simulink model "Balance_DualGyro_150302"  (R2014a)
settings: Solver=FixedStepDiscrete  SolverMode=SingleTasking  StartTime=0.0  StopTime=inf  FixedStep=TS  RelTol=1e-3
undefined symbols (not defined in the file or in its folder): DiscIntNeverNeededParam, ES, GS, KLQR, Rw, TS
libraries: arduinolib x7, simulink x4
settings Model: FPTRunName=FPA_Reference  SimulationMode=external  ExtModeTrigDuration=2  Creator=Alec  LastModifiedBy=Brian
settings OptimizationCC: ExpressionDepthLimit=2147483647  OptimizeModelRefInitCode=on  LifeSpan=1
settings DebuggingCC: UnderspecifiedInitializationDetection=Classic  SolverPrmCheckMsg=none  StateNameClashWarn=warning
settings HardwareCC: ProdBitPerInt=16  ProdBitPerPointer=8  ProdIntDivRoundTo=Zero  ProdEndianess=LittleEndian  ProdWordSize=8  ProdHWDeviceType=Atmel->AVR
settings RTWCC: SystemTargetFile=realtime.tlc  GenerateMakefile=off  TemplateMakefile=realtime.tmf  Description=Real-Time Toolbox  RTWVerbose=off  ProcessScript=realtime_make_rtw_hook
settings CodeAppCC: CustomSymbolStrType=$N$R$M  InternalIdentifier=Classic
settings STFCustomTargetCC: TargetLibSuffix=.a  GenerateSampleERTMain=on  ConcurrentExecutionCompliant=off  GeneratePreprocessorConditionals=Use local settings  ERTCustomFileBanners=on  SupportNonInlinedSFcns=off  SupportVariableSizeSignals=on  MATLABClassNameForMDSCustomization=Simulink.SoftwareTarget.ERTCustomization  GRTInterface=off  SystemTargetFile=realtime.tlc
settings ERTTargetCC: CombineOutputUpdateFcns=off  SupportContinuousTime=on  SupportVariableSizeSignals=on  ExtModeTransport=3  ExtModeMexFile=ext_serial_win32_comm  ExtModeMexArgs=0 6 115200  ERTSrcFileBannerTemplate=realtime_code_template.cgt  ERTHdrFileBannerTemplate=realtime_code_template.cgt  ERTDataSrcFileTemplate=realtime_code_template.cgt  ERTDataHdrFileTemplate=realtime_code_template.cgt  ERTCustomFileTemplate=realtime_file_process.tlc

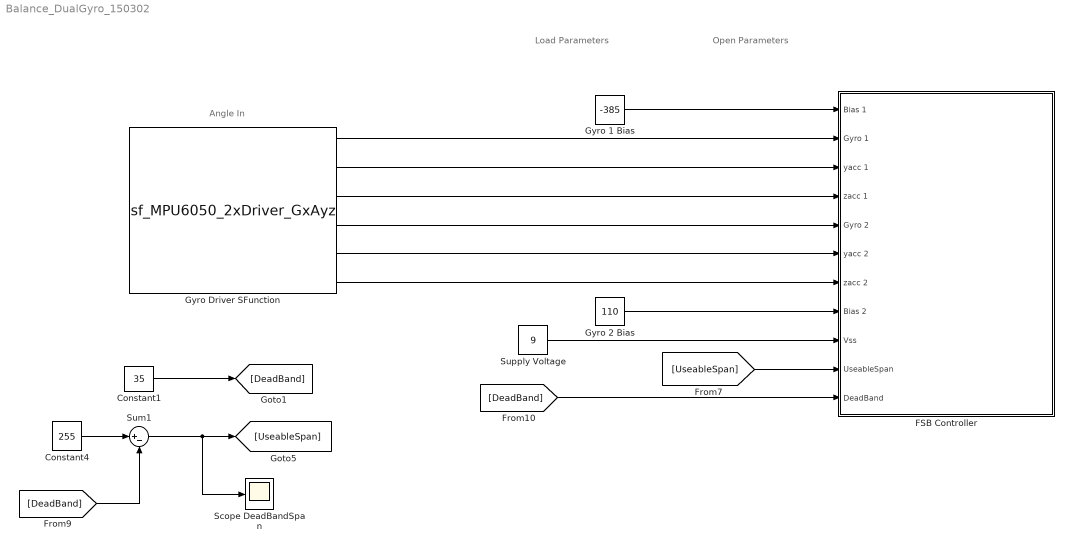
== system Balance_DualGyro_150302 ==
  note: Load Parameters
  note: Open Parameters
  note: Angle In
  Constant1 : Constant  Value=35
  Constant4 : Constant  Value=255
  FSB Controller : Subsystem
  Gyro 1 Bias : Constant  Value=-385
  Gyro 2 Bias : Constant  Value=110
  Gyro Driver SFunction : S-Function  InitFcn=try, set_param(gcb,'FunctionName','sf_MPU6050_2xDriver_GxAyz'), end  FunctionName=sf_MPU6050_2xDriver_GxAyz  SFunctionModules=sf_MPU6050_2xDriver_GxAyz_wrapper  EnableBusSupport=off  mask(S-Function Builder){}
      mask help: Simulink:masks:SFunctionBuilder_MD
      mask init:
      | val = [[.9  0.75 0.75 1 1 .9 .9 1]',[1 1 0.75 0.75 .9 .9 1 .9]'];try , sys = get_param(gcb,'SfunBuilderFcnName');if isempty(sys), sys = get_param(gcb,'FunctionName'); end,catch, sys = get_param(gcb,'FunctionName'); end
      settings: CopyFcn=set_param(gcbh,'LinkStatus','none')  PreSaveFcn=try, set_param(gcb,'FunctionName','sf_MPU6050_2xDriver_GxAyz'), end  OpenFcn=sfunctionwizard(gcbh)
      mask Display: plot(val(:,1),val(:,2)),disp(sys), port_label('output',1,'x_vel'), port_label('output',2,'y_acc'), port_label('output',3,'z_acc'), port_label('output',4,'x_vel_2'), port_label('output',5,'y_acc_2'), port_label('output',6,'z_acc_2')
  Scope DeadBandSpan : Scope
      settings: YMin=205  YMax=205  SaveName=ScopeData5
  Sum1 : Sum  Inputs=|+-
  Supply Voltage : Constant  Value=9
  wires:
  Gyro Driver SFunction/3 -> FSB Controller/4("zacc 1 ")
  Gyro 1 Bias/1 -> FSB Controller/1(Bias 1)
  Constant1/1 -> [DeadBand]
  Constant4/1 -> Sum1/1
  [DeadBand] -> Sum1/2
  Sum1/1 -> Scope DeadBandSpan/1, [UseableSpan]
  [DeadBand] -> FSB Controller/11(DeadBand)
  Supply Voltage/1 -> FSB Controller/9(Vss)
  Gyro Driver SFunction/2 -> FSB Controller/3("yacc 1 ")
  [UseableSpan] -> FSB Controller/10(UseableSpan)
  Gyro 2 Bias/1 -> FSB Controller/8(Bias 2)
  Gyro Driver SFunction/4 -> FSB Controller/5(Gyro 2)
  Gyro Driver SFunction/5 -> FSB Controller/6(yacc 2)
  Gyro Driver SFunction/6 -> FSB Controller/7(zacc 2)
  Gyro Driver SFunction/1 -> FSB Controller/2(Gyro 1)

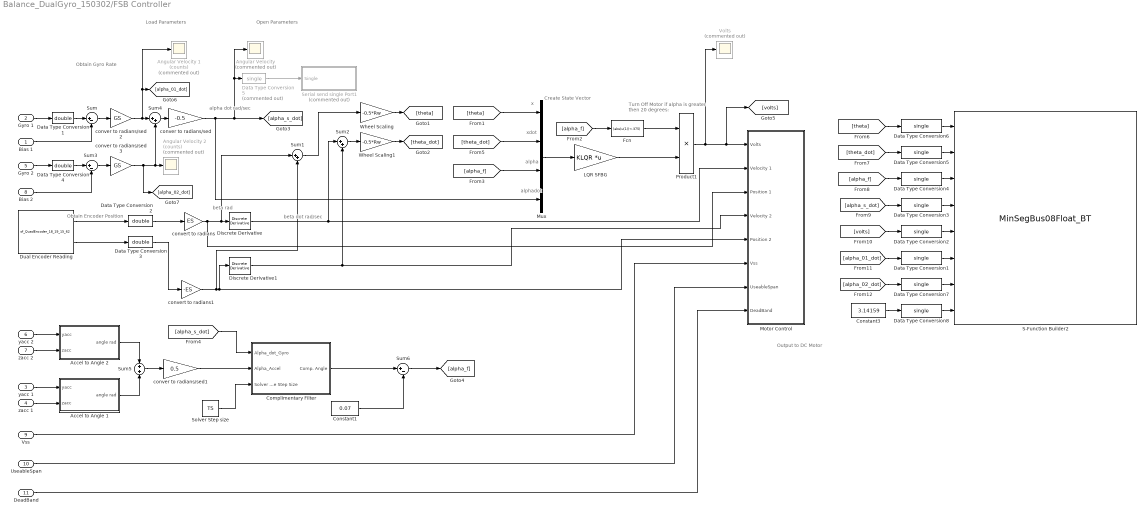
== system Balance_DualGyro_150302/FSB Controller ==
  note: Turn Off Motor if alpha is
      | greater then 20 degrees:
  note: Output to DC Motor
  note: Create State Vector
  note: Obtain Encoder Position
  note: Obtain Gyro Rate
  note: xdot
  note: x
  note: beta
      | rad
  note: alpha dot
      | rad/sec
  note: beta dot
      | rad/sec
  note: alpha
  note: alphadot
  note: Load Parameters
  note: Open Parameters
  Bias 1 : Inport
  Gyro 1 : Inport  Port=2
  "yacc 1 " : Inport  Port=3
  "zacc 1 " : Inport  Port=4
  Gyro 2 : Inport  Port=5
  yacc 2 : Inport  Port=6
  zacc 2 : Inport  Port=7
  Bias 2 : Inport  Port=8
  Vss : Inport  Port=9
  UseableSpan : Inport  Port=10
  DeadBand : Inport  Port=11
  Accel to Angle 1 : Subsystem
  Accel to Angle 2 : Subsystem
  Angular Velocity : Scope  Commented=on
      settings: YMin=-0.25  YMax=0.175
  Angular Velocity 1 (counts) : Scope  Commented=on
      settings: YMin=100  YMax=500  SaveName=ScopeData13
  Angular Velocity 2 (counts) : Scope  Commented=on
      settings: YMin=100  YMax=500  SaveName=ScopeData14
  Complimentary Filter : Subsystem
  Constant1 : Constant  Value=0.07
  Constant3 : Constant  Value=3.14159
  Data Type Conversion{1..4} (4 alike) : DataTypeConversion  OutDataTypeStr=double
  Data Type Conversion5 : DataTypeConversion  Commented=on  OutDataTypeStr=single
  Data Type Conversion{1..8} (8 alike) : DataTypeConversion  OutDataTypeStr=single
  Discrete Derivative : simulink/Discrete/Discrete Derivative  gainval=1.0  ICPrevScaledInput=0.0  InputProcessing=Inherited  OutMin=[]  OutMax=[]  OutDataType=fixdt(1, 16)  OutScaling=2^-10  DoSatur=off
  Discrete Derivative1 : simulink/Discrete/Discrete Derivative  gainval=1.0  ICPrevScaledInput=0.0  InputProcessing=Inherited  OutMin=[]  OutMax=[]  OutDataType=fixdt(1, 16)  OutScaling=2^-10  DoSatur=off
  Dual Encoder Reading : S-Function  InitFcn=try, set_param(gcb,'FunctionName','sf_QuadEncoder_18_19_15_62'), end  FunctionName=sf_QuadEncoder_18_19_15_62  Parameters=uint8([0 1]),uint8([18 62]),uint8([19 15])  SFunctionModules=sf_QuadEncoder_18_19_15_62_wrapper  EnableBusSupport=off  mask(S-Function Builder){}
      mask init: same as Balance_DualGyro_150302/Gyro Driver SFunction
      settings: CopyFcn=set_param(gcbh,'LinkStatus','none')  PreSaveFcn=try, set_param(gcb,'FunctionName','sf_QuadEncoder_18_19_15_62'), end  OpenFcn=sfunctionwizard(gcbh)
      mask Display: plot(val(:,1),val(:,2)),disp(sys), port_label('output',1,'pos1'), port_label('output',2,'pos2')
  Fcn : Fcn  Expr=(abs(u(1))<.375)
  LQR SFBG : Gain  Gain=KLQR  Multiplication=Matrix(K*u)
  Motor Control : Subsystem
  Mux : Mux
  Product1 : Product  RndMeth=Zero
  S-Function Builder2 : S-Function  InitFcn=try, set_param(gcb,'FunctionName','MinSegBus08Float_BT'), end  FunctionName=MinSegBus08Float_BT  Parameters=int8(4)  SFunctionModules=MinSegBus08Float_BT_wrapper  EnableBusSupport=off  mask(S-Function Builder){}
      mask help: Simulink:masks:SFunctionBuilder_MD
      mask init: same as Balance_DualGyro_150302/Gyro Driver SFunction
      settings: CopyFcn=set_param(gcbh,'LinkStatus','none')  PreSaveFcn=try, set_param(gcb,'FunctionName','MinSegBus08Float_BT'), end  OpenFcn=sfunctionwizard(gcbh)
      mask Display: plot(val(:,1),val(:,2)),disp(sys), port_label('input',1,'float_01'), port_label('input',2,'float_02'), port_label('input',3,'float_03'), port_label('input',4,'float_04'), port_label('input',5,'float_05'), port_label('input',6,'float_06'), port_label('input',7,'float_07'), port_label('input',8,'float_08')
  Serial send single Port1 : Subsystem  Commented=on  TreatAsAtomicUnit=on
  Solver Step size : Constant  Value=TS
  Sum : Sum  Inputs=|+-
  Sum1 : Sum  Inputs=|++
  Sum2 : Sum  Inputs=|++
  Sum3 : Sum  Inputs=|+-
  Sum4 : Sum  Inputs=|++
  Sum5 : Sum  Inputs=+|+
  Sum6 : Sum  Inputs=|+-
  Volts : Scope  Commented=on
      settings: YMin=-12.5  YMax=10  SaveName=ScopeData7
  Wheel Scaling : Gain  Gain=-0.5*Rw
  Wheel Scaling1 : Gain  Gain=-0.5*Rw
  conver to radians/sed : Gain  Gain=-0.5
  conver to radians/sed1 : Gain  Gain=0.5
  conver to radians/sed2 : Gain  Gain=GS
  conver to radians/sed3 : Gain  Gain=GS
  convert to radians : Gain  Gain=ES  OutDataTypeStr=double
  convert to radians1 : Gain  Gain=-ES  OutDataTypeStr=double
  wires:
  Bias 1/1 -> Sum/2
  convert to radians/1 -> Motor Control/3(Position 1), Sum1/1, Discrete Derivative/1
  Data Type Conversion1/1 -> Sum/1
  Gyro 1/1 -> Data Type Conversion1/1
  [alpha_f] -> Fcn/1
  conver to radians/sed/1 -> Data Type Conversion5/1, Angular Velocity/1, [alpha_s_dot], Mux/4
  "yacc 1 "/1 -> Accel to Angle 1/1(yacc)
  "zacc 1 "/1 -> Accel to Angle 1/2(zacc)
  [alpha_f] -> Mux/3
  LQR SFBG/1 -> Product1/2
  Fcn/1 -> Product1/1
  Mux/1 -> LQR SFBG/1
  [alpha_s_dot] -> Complimentary Filter/1(Alpha_dot_Gyro)
  Solver Step size/1 -> Complimentary Filter/3(Solver Time Step Size)
  convert to radians1/1 -> Sum1/2, Discrete Derivative1/1, Motor Control/5(Position 2)
  Dual Encoder Reading/1 -> Data Type Conversion2/1
  Data Type Conversion2/1 -> convert to radians/1
  [theta] -> Mux/1
  Dual Encoder Reading/2 -> Data Type Conversion3/1
  Data Type Conversion3/1 -> convert to radians1/1
  Discrete Derivative1/1 -> Motor Control/4(Velocity 2), Sum2/2
  Vss/1 -> Motor Control/6(Vss)
  Sum2/1 -> Wheel Scaling1/1
  Discrete Derivative/1 -> Motor Control/2(Velocity 1), Sum2/1
  Data Type Conversion5/1 -> Serial send single Port1/1(Single)
  UseableSpan/1 -> Motor Control/7(UseableSpan)
  DeadBand/1 -> Motor Control/8(DeadBand)
  Product1/1 -> Volts/1, [volts], Motor Control/1(Volts)
  yacc 2/1 -> Accel to Angle 2/1(yacc)
  zacc 2/1 -> Accel to Angle 2/2(zacc)
  Gyro 2/1 -> Data Type Conversion4/1
  Bias 2/1 -> Sum3/2
  Data Type Conversion4/1 -> Sum3/1
  Sum4/1 -> conver to radians/sed/1
  Sum/1 -> conver to radians/sed2/1
  Sum3/1 -> conver to radians/sed3/1
  Accel to Angle 1/1(angle rad) -> Sum5/2
  Accel to Angle 2/1(angle rad) -> Sum5/1
  Sum5/1 -> conver to radians/sed1/1
  conver to radians/sed1/1 -> Complimentary Filter/2(Alpha_Accel)
  Sum1/1 -> Wheel Scaling/1
  Wheel Scaling/1 -> [theta]
  Wheel Scaling1/1 -> [theta_dot]
  [theta_dot] -> Mux/2
  Data Type Conversion1/1 -> S-Function Builder2/6
  [volts] -> Data Type Conversion2/1
  Data Type Conversion2/1 -> S-Function Builder2/5
  Data Type Conversion3/1 -> S-Function Builder2/4
  [alpha_s_dot] -> Data Type Conversion3/1
  [theta] -> Data Type Conversion6/1
  Data Type Conversion6/1 -> S-Function Builder2/1
  Data Type Conversion5/1 -> S-Function Builder2/2
  [theta_dot] -> Data Type Conversion5/1
  [alpha_f] -> Data Type Conversion4/1
  Data Type Conversion4/1 -> S-Function Builder2/3
  Data Type Conversion7/1 -> S-Function Builder2/7
  Data Type Conversion8/1 -> S-Function Builder2/8
  Constant3/1 -> Data Type Conversion8/1
  conver to radians/sed2/1 -> Angular Velocity 1 (counts)/1, [alpha_01_dot], Sum4/1
  conver to radians/sed3/1 -> [alpha_02_dot], Angular Velocity 2 (counts)/1, Sum4/2
  [alpha_01_dot] -> Data Type Conversion1/1
  [alpha_02_dot] -> Data Type Conversion7/1
  Complimentary Filter/1(Comp. Angle) -> Sum6/1
  Sum6/1 -> [alpha_f]
  Constant1/1 -> Sum6/2

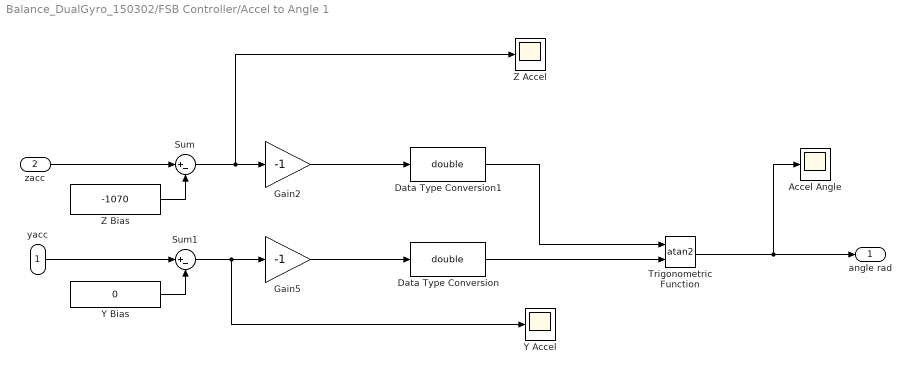
== system Balance_DualGyro_150302/FSB Controller/Accel to Angle 1 ==
  yacc : Inport
  zacc : Inport  Port=2
  Accel Angle : Scope
      settings: YMin=-0.0025  YMax=0.003  SaveName=ScopeData9
  Data Type Conversion : DataTypeConversion  OutDataTypeStr=double
  Data Type Conversion1 : DataTypeConversion  OutDataTypeStr=double
  Gain2 : Gain  Gain=-1
  Gain5 : Gain  Gain=-1
  Sum : Sum  Inputs=|+-
  Sum1 : Sum  Inputs=|+-
  Trigonometric Function : Trigonometry  Operator=atan2
  "Y Accel " : Scope
      settings: YMin=-16380  YMax=-16320  SaveName=ScopeData8
  Y Bias : Constant  Value=0
  Z Accel : Scope
      settings: YMin=-1500  YMax=1750  SaveName=ScopeData3
  Z Bias : Constant  Value=-1070
  angle rad : Outport
  wires:
  Z Bias/1 -> Sum/2
  Y Bias/1 -> Sum1/2
  Trigonometric Function/1 -> Accel Angle/1, angle rad/1
  Data Type Conversion1/1 -> Trigonometric Function/1
  Data Type Conversion/1 -> Trigonometric Function/2
  zacc/1 -> Sum/1
  yacc/1 -> Sum1/1
  Gain2/1 -> Data Type Conversion1/1
  Sum/1 -> Z Accel/1, Gain2/1
  Sum1/1 -> "Y Accel "/1, Gain5/1
  Gain5/1 -> Data Type Conversion/1

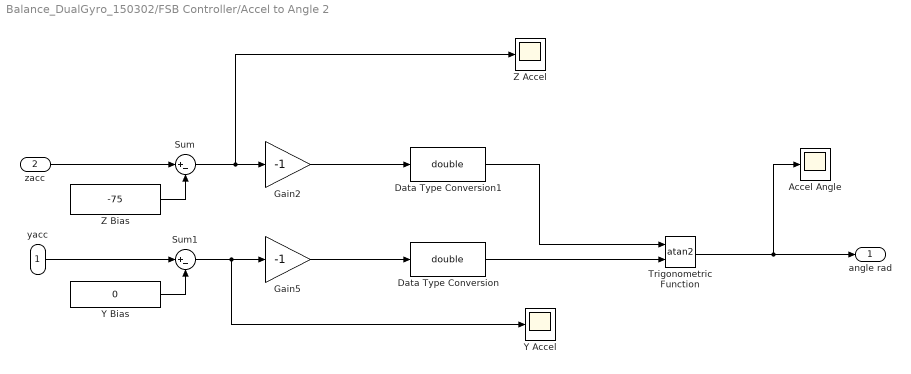
== system Balance_DualGyro_150302/FSB Controller/Accel to Angle 2 ==
  yacc : Inport
  zacc : Inport  Port=2
  Accel Angle : Scope
      settings: YMin=-0.00275  YMax=0.0015  SaveName=ScopeData9
  Data Type Conversion : DataTypeConversion  OutDataTypeStr=double
  Data Type Conversion1 : DataTypeConversion  OutDataTypeStr=double
  Gain2 : Gain  Gain=-1
  Gain5 : Gain  Gain=-1
  Sum : Sum  Inputs=|+-
  Sum1 : Sum  Inputs=|+-
  Trigonometric Function : Trigonometry  Operator=atan2
  "Y Accel " : Scope
      settings: YMin=-16405  YMax=-16350  SaveName=ScopeData8
  Y Bias : Constant  Value=0
  Z Accel : Scope
      settings: YMin=-35  YMax=45  SaveName=ScopeData3
  Z Bias : Constant  Value=-75
  angle rad : Outport
  wires:
  Z Bias/1 -> Sum/2
  Y Bias/1 -> Sum1/2
  Trigonometric Function/1 -> Accel Angle/1, angle rad/1
  Data Type Conversion1/1 -> Trigonometric Function/1
  Data Type Conversion/1 -> Trigonometric Function/2
  zacc/1 -> Sum/1
  yacc/1 -> Sum1/1
  Gain2/1 -> Data Type Conversion1/1
  Sum/1 -> Z Accel/1, Gain2/1
  Sum1/1 -> "Y Accel "/1, Gain5/1
  Gain5/1 -> Data Type Conversion/1

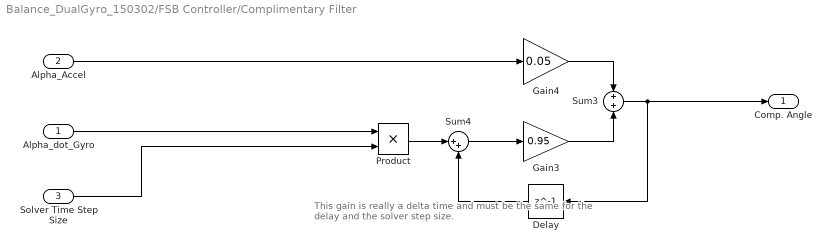
== system Balance_DualGyro_150302/FSB Controller/Complimentary Filter ==
  note: This gain is really a delta time and must be the same for
      | the delay and the solver step size.
  Alpha_dot_Gyro : Inport
  Alpha_Accel : Inport  Port=2
  Solver Time Step Size : Inport  Port=3
  Delay : Delay  DelayLength=1  InitialCondition=0
  Gain3 : Gain  Gain=0.95
  Gain4 : Gain  Gain=0.05
  Product : Product
  Sum3 : Sum
  Sum4 : Sum  Inputs=|++
  Comp. Angle : Outport
  wires:
  Gain3/1 -> Sum3/2
  Gain4/1 -> Sum3/1
  Sum3/1 -> Comp. Angle/1, Delay/1
  Sum4/1 -> Gain3/1
  Delay/1 -> Sum4/2
  Product/1 -> Sum4/1
  Alpha_Accel/1 -> Gain4/1
  Alpha_dot_Gyro/1 -> Product/1
  Solver Time Step Size/1 -> Product/2

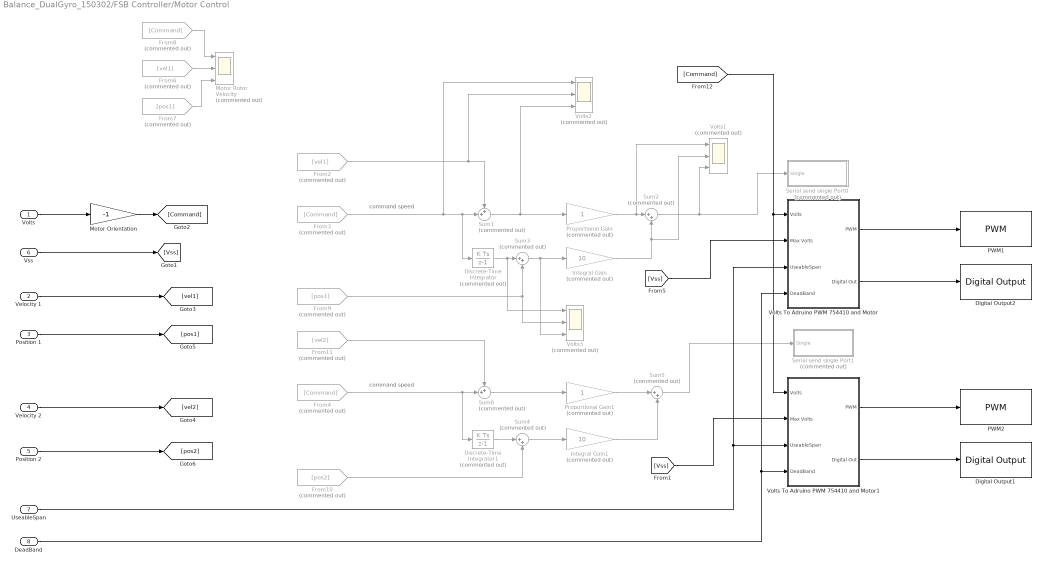
== system Balance_DualGyro_150302/FSB Controller/Motor Control ==
  note: command speed
  note: command speed
  Volts : Inport
  Velocity 1 : Inport  Port=2
  Position 1 : Inport  Port=3
  Velocity 2 : Inport  Port=4
  Position 2 : Inport  Port=5
  Vss : Inport  Port=6
  UseableSpan : Inport  Port=7
  DeadBand : Inport  Port=8
  Digital Output1 : arduinolib/Digital Output  pinNumber=2
  Digital Output2 : arduinolib/Digital Output  pinNumber=6
  Discrete-Time Integrator : DiscreteIntegrator  Commented=on  SampleTime=-1  OutDataTypeStr=double  ICPrevOutput=DiscIntNeverNeededParam  ICPrevScaledInput=DiscIntNeverNeededParam
  Discrete-Time Integrator1 : DiscreteIntegrator  Commented=on  SampleTime=-1  OutDataTypeStr=double  ICPrevOutput=DiscIntNeverNeededParam  ICPrevScaledInput=DiscIntNeverNeededParam
  From10 : From  Commented=on  GotoTag=pos2
  From11 : From  Commented=on  GotoTag=vel2
  From2 : From  Commented=on  GotoTag=vel1
  From3 : From  Commented=on  GotoTag=Command
  From4 : From  Commented=on  GotoTag=Command
  From6 : From  Commented=on  GotoTag=vel1
  From7 : From  Commented=on  GotoTag=pos1
  From8 : From  Commented=on  GotoTag=Command
  From9 : From  Commented=on  GotoTag=pos1
  Integral Gain : Gain  Commented=on  Gain=10
  Integral Gain1 : Gain  Commented=on  Gain=10
  Motor Orientation : Gain  Gain=-1
  Motor Rotor Velocity : Scope  Commented=on  NumInputPorts=3
      settings: YMin=-1~-8~3  YMax=1~7~6.25
  PWM1 : arduinolib/PWM  pinNumber=8
  PWM2 : arduinolib/PWM  pinNumber=5
  Proportional Gain : Gain  Commented=on
  Proportional Gain1 : Gain  Commented=on
  Serial send single Port0 : Subsystem  Commented=on  TreatAsAtomicUnit=on
  Serial send single Port1 : Subsystem  Commented=on  TreatAsAtomicUnit=on
  Sum1 : Sum  Commented=on  Inputs=++|
  Sum{2..5} (4 alike) : Sum  Commented=on  Inputs=|++
  Sum6 : Sum  Commented=on  Inputs=++|
  Volts To Adruino PWM 754410 and Motor : Subsystem
  Volts To Adruino PWM 754410 and Motor1 : Subsystem
  Volts1 : Scope  Commented=on  NumInputPorts=3
      settings: YMin=-12.5~-5~-5  YMax=10~5~5  SaveName=ScopeData10
  Volts2 : Scope  Commented=on  NumInputPorts=3
      settings: YMin=-12.5~-5~-5  YMax=10~5~5  SaveName=ScopeData11
  Volts3 : Scope  Commented=on  NumInputPorts=3
      settings: YMin=-12.5~-5~-5  YMax=10~5~5  SaveName=ScopeData12
  wires:
  Volts/1 -> Motor Orientation/1
  Sum5/1 -> Serial send single Port1/1(Single)
  Sum6/1 -> Proportional Gain1/1
  From11/1 -> Sum6/1
  Motor Orientation/1 -> [Command]
  Velocity 2/1 -> [vel2]
  Vss/1 -> [Vss]
  [Vss] -> Volts To Adruino PWM 754410 and Motor1/2(Max Volts)
  Sum1/1 -> Volts2/3, Proportional Gain/1
  From2/1 -> Volts2/2, Sum1/1
  Velocity 1/1 -> [vel1]
  Position 1/1 -> [pos1]
  Position 2/1 -> [pos2]
  [Vss] -> Volts To Adruino PWM 754410 and Motor/2(Max Volts)
  From7/1 -> Motor Rotor Velocity/3
  From6/1 -> Motor Rotor Velocity/2
  From8/1 -> Motor Rotor Velocity/1
  Proportional Gain/1 -> Volts1/1, Sum2/1
  Sum2/1 -> Volts1/3, Serial send single Port0/1(Single)
  Discrete-Time Integrator/1 -> Volts3/1, Sum3/1
  Sum3/1 -> Volts3/3, Integral Gain/1
  From3/1 -> Volts2/1, Discrete-Time Integrator/1, Sum1/2
  From9/1 -> Sum3/2, Volts3/2
  Discrete-Time Integrator1/1 -> Sum4/1
  Sum4/1 -> Integral Gain1/1
  From4/1 -> Discrete-Time Integrator1/1, Sum6/2
  From10/1 -> Sum4/2
  Proportional Gain1/1 -> Sum5/1
  Integral Gain1/1 -> Sum5/2
  Volts To Adruino PWM 754410 and Motor/1(PWM) -> PWM1/1
  Volts To Adruino PWM 754410 and Motor/2(Digital Out) -> Digital Output2/1
  Volts To Adruino PWM 754410 and Motor1/1(PWM) -> PWM2/1
  Volts To Adruino PWM 754410 and Motor1/2(Digital Out) -> Digital Output1/1
  UseableSpan/1 -> Volts To Adruino PWM 754410 and Motor/3(UseableSpan), Volts To Adruino PWM 754410 and Motor1/3(UseableSpan)
  DeadBand/1 -> Volts To Adruino PWM 754410 and Motor1/4(DeadBand), Volts To Adruino PWM 754410 and Motor/4(DeadBand)
  Integral Gain/1 -> Volts1/2, Sum2/2
  [Command] -> Volts To Adruino PWM 754410 and Motor/1(Volts), Volts To Adruino PWM 754410 and Motor1/1(Volts)

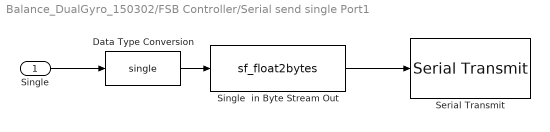
== system Balance_DualGyro_150302/FSB Controller/Serial send single Port1 ==
  Single : Inport
  Data Type Conversion : DataTypeConversion  OutDataTypeStr=single
  Serial Transmit : arduinolib/Serial Transmit  portNumber=0
  Single  in Byte Stream Out : S-Function  InitFcn=try, set_param(gcb,'FunctionName','sf_float2bytes'), end  FunctionName=sf_float2bytes  SFunctionModules=sf_float2bytes_wrapper  EnableBusSupport=off  mask(S-Function Builder){}
      mask init: same as Balance_DualGyro_150302/Gyro Driver SFunction
      settings: CopyFcn=set_param(gcb,'LinkStatus','none')  PreSaveFcn=try, set_param(gcb,'FunctionName','sf_float2bytes'), end  OpenFcn=sfunctionwizard(gcbh)
      mask Display: plot(val(:,1),val(:,2)),disp(sys), port_label('input',1,'fin'), port_label('output',1,'bout')
  wires:
  Single/1 -> Data Type Conversion/1
  Data Type Conversion/1 -> Single  in Byte Stream Out/1
  Single  in Byte Stream Out/1 -> Serial Transmit/1

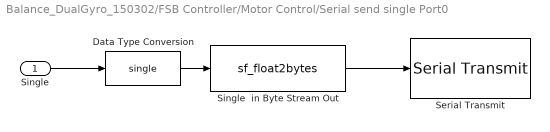
== system Balance_DualGyro_150302/FSB Controller/Motor Control/Serial send single Port0 ==
  Single : Inport
  Data Type Conversion : DataTypeConversion  OutDataTypeStr=single
  Serial Transmit : arduinolib/Serial Transmit  portNumber=0
  Single  in Byte Stream Out : S-Function  InitFcn=try, set_param(gcb,'FunctionName','sf_float2bytes'), end  FunctionName=sf_float2bytes  SFunctionModules=sf_float2bytes_wrapper  EnableBusSupport=off  mask(S-Function Builder){}
      mask init: same as Balance_DualGyro_150302/Gyro Driver SFunction
      settings: CopyFcn=set_param(gcb,'LinkStatus','none')  PreSaveFcn=try, set_param(gcb,'FunctionName','sf_float2bytes'), end  OpenFcn=sfunctionwizard(gcbh)
      mask Display: plot(val(:,1),val(:,2)),disp(sys), port_label('input',1,'fin'), port_label('output',1,'bout')
  wires:
  Single/1 -> Data Type Conversion/1
  Data Type Conversion/1 -> Single  in Byte Stream Out/1
  Single  in Byte Stream Out/1 -> Serial Transmit/1

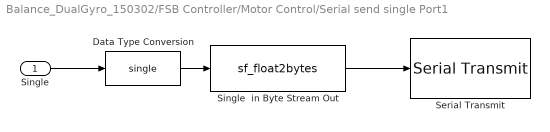
== system Balance_DualGyro_150302/FSB Controller/Motor Control/Serial send single Port1 ==
  Single : Inport
  Data Type Conversion : DataTypeConversion  OutDataTypeStr=single
  Serial Transmit : arduinolib/Serial Transmit  portNumber=0
  Single  in Byte Stream Out : S-Function  InitFcn=try, set_param(gcb,'FunctionName','sf_float2bytes'), end  FunctionName=sf_float2bytes  SFunctionModules=sf_float2bytes_wrapper  EnableBusSupport=off  mask(S-Function Builder){}
      mask init: same as Balance_DualGyro_150302/Gyro Driver SFunction
      settings: CopyFcn=set_param(gcb,'LinkStatus','none')  PreSaveFcn=try, set_param(gcb,'FunctionName','sf_float2bytes'), end  OpenFcn=sfunctionwizard(gcbh)
      mask Display: plot(val(:,1),val(:,2)),disp(sys), port_label('input',1,'fin'), port_label('output',1,'bout')
  wires:
  Single/1 -> Data Type Conversion/1
  Data Type Conversion/1 -> Single  in Byte Stream Out/1
  Single  in Byte Stream Out/1 -> Serial Transmit/1

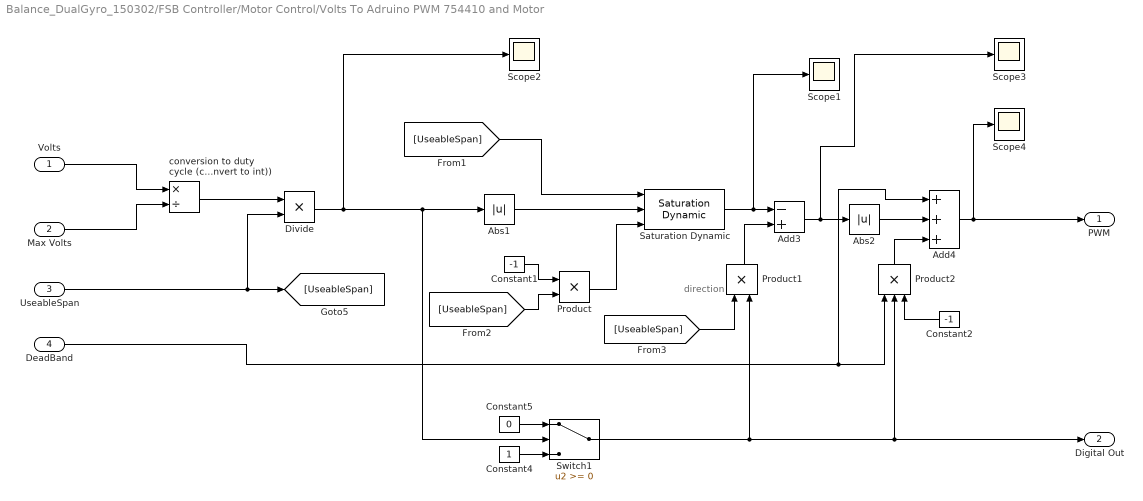
== system Balance_DualGyro_150302/FSB Controller/Motor Control/Volts To Adruino PWM 754410 and Motor ==
  note: direction
  Volts : Inport
  Max Volts : Inport  Port=2
  UseableSpan : Inport  Port=3
  DeadBand : Inport  Port=4
  Abs1 : Abs
  Abs2 : Abs
  Add3 : Sum  Inputs=-+
  Add4 : Sum  Inputs=+++
  Constant1 : Constant  Value=-1
  Constant2 : Constant  Value=-1
  Constant4 : Constant
  Constant5 : Constant  Value=0
  Divide : Product  Inputs=**
  Product : Product
  Product1 : Product
  Product2 : Product  Inputs=3
  Saturation Dynamic : simulink/Discontinuities/Saturation Dynamic  OutMin=[]  OutMax=[]  OutDataTypeStr=Inherit: Same as second input  OutDataType=fixdt(1, 16)  OutScaling=2^-10  DoSatur=off
  Scope{1..4} (4 alike) : Scope
      Scope1 settings: YMin=41  YMax=41  SaveName=ScopeData4
      Scope2 settings: YMin=38.95  YMax=43.05
      Scope3 settings: YMin=155.8  YMax=172.2  SaveName=ScopeData6
      Scope4 settings: YMin=250.8  YMax=277.2  SaveName=ScopeData7
  Switch1 : Switch
  conversion to duty cycle (convert to int)) : Product  Inputs=*/  OutDataTypeStr=double
  PWM : Outport
  Digital Out : Outport  Port=2
  wires:
  Abs1/1 -> Saturation Dynamic/2
  Saturation Dynamic/1 -> Scope1/1, Add3/1
  Add3/1 -> Scope3/1, Abs2/1
  Product1/1 -> Add3/2
  Constant4/1 -> Switch1/3
  Constant5/1 -> Switch1/1
  Switch1/1 -> Product1/2, Digital Out/1, Product2/2
  Abs2/1 -> Add4/2
  DeadBand/1 -> Add4/1, Product2/1
  Max Volts/1 -> conversion to duty cycle (convert to int))/2
  Product2/1 -> Add4/3
  Volts/1 -> conversion to duty cycle (convert to int))/1
  conversion to duty cycle (convert to int))/1 -> Divide/1
  [UseableSpan] -> Saturation Dynamic/1
  [UseableSpan] -> Product/2
  Constant1/1 -> Product/1
  Product/1 -> Saturation Dynamic/3
  [UseableSpan] -> Product1/1
  Divide/1 -> Scope2/1, Abs1/1, Switch1/2
  UseableSpan/1 -> Divide/2, [UseableSpan]
  Add4/1 -> PWM/1, Scope4/1
  Constant2/1 -> Product2/3

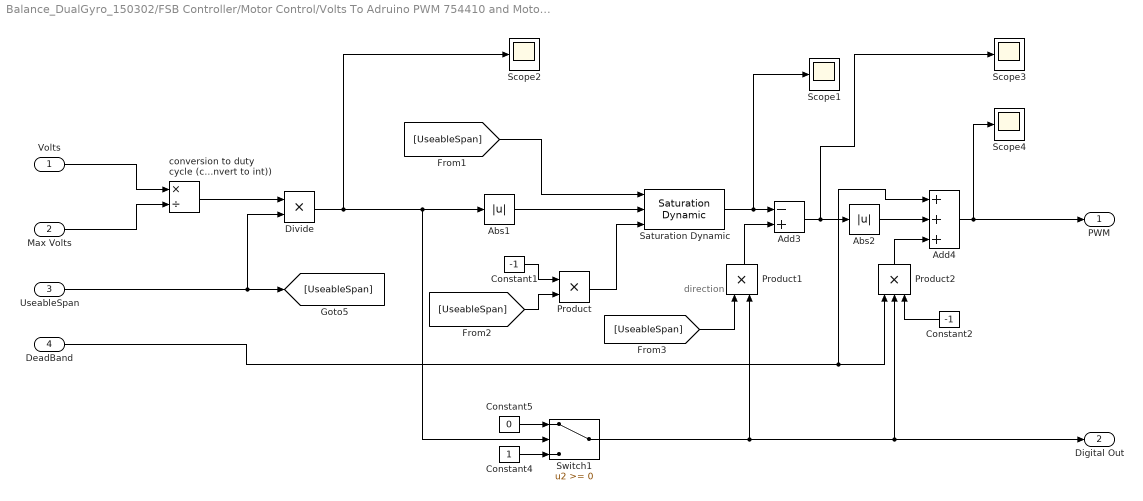
== system Balance_DualGyro_150302/FSB Controller/Motor Control/Volts To Adruino PWM 754410 and Motor1 ==
  note: direction
  Volts : Inport
  Max Volts : Inport  Port=2
  UseableSpan : Inport  Port=3
  DeadBand : Inport  Port=4
  Abs1 : Abs
  Abs2 : Abs
  Add3 : Sum  Inputs=-+
  Add4 : Sum  Inputs=+++
  Constant1 : Constant  Value=-1
  Constant2 : Constant  Value=-1
  Constant4 : Constant
  Constant5 : Constant  Value=0
  Divide : Product  Inputs=**
  Product : Product
  Product1 : Product
  Product2 : Product  Inputs=3
  Saturation Dynamic : simulink/Discontinuities/Saturation Dynamic  OutMin=[]  OutMax=[]  OutDataTypeStr=Inherit: Same as second input  OutDataType=fixdt(1, 16)  OutScaling=2^-10  DoSatur=off
  Scope{1..4} (4 alike) : Scope
      Scope1 settings: YMin=41  YMax=41  SaveName=ScopeData4
      Scope2 settings: YMin=38.95  YMax=43.05
      Scope3 settings: YMin=155.8  YMax=172.2  SaveName=ScopeData6
      Scope4 settings: YMin=250.8  YMax=277.2  SaveName=ScopeData7
  Switch1 : Switch
  conversion to duty cycle (convert to int)) : Product  Inputs=*/  OutDataTypeStr=double
  PWM : Outport
  Digital Out : Outport  Port=2
  wires:
  Abs1/1 -> Saturation Dynamic/2
  Saturation Dynamic/1 -> Scope1/1, Add3/1
  Add3/1 -> Scope3/1, Abs2/1
  Product1/1 -> Add3/2
  Constant4/1 -> Switch1/3
  Constant5/1 -> Switch1/1
  Switch1/1 -> Product1/2, Digital Out/1, Product2/2
  Abs2/1 -> Add4/2
  DeadBand/1 -> Add4/1, Product2/1
  Max Volts/1 -> conversion to duty cycle (convert to int))/2
  Product2/1 -> Add4/3
  Volts/1 -> conversion to duty cycle (convert to int))/1
  conversion to duty cycle (convert to int))/1 -> Divide/1
  [UseableSpan] -> Saturation Dynamic/1
  [UseableSpan] -> Product/2
  Constant1/1 -> Product/1
  Product/1 -> Saturation Dynamic/3
  [UseableSpan] -> Product1/1
  Divide/1 -> Scope2/1, Abs1/1, Switch1/2
  UseableSpan/1 -> Divide/2, [UseableSpan]
  Add4/1 -> PWM/1, Scope4/1
  Constant2/1 -> Product2/3
